simulink model "ex11"  (Simulink 6.3)
settings: Solver=VariableStepDiscrete  StartTime=0.0  StopTime=10.0  RelTol=1e-3
values from neighbouring files (symbols this model uses):
  BitRate = 100000    [ex11sim.m]
  Lc = 7    [ex11sim.m]
libraries: commcnvcod2 x3, commdigbbndpm2 x2, commsink2 x2, commchan3 x1, commrandsrc2 x1, simulink x1
settings Model: LastModifiedBy=lxy  StrictBusMsg=None
settings OptimizationCC: InlineInvariantSignals=on

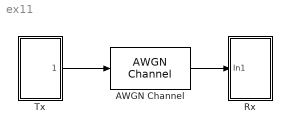
== system ex11 ==
  AWGN Channel : commchan3/AWGN Channel  seed=67  noiseMode="Signal to noise ratio  (Eb/No)"  EbNodB=SNR  EsNodB=10  SNRdB=10  bitsPerSym=1  Ps=1  Tsym=1/BitRate  variance=1
  Rx : Subsystem
  Tx : Subsystem
  wires:
  Tx/1(Signal) -> AWGN Channel/1
  AWGN Channel/1 -> Rx/1(In1)

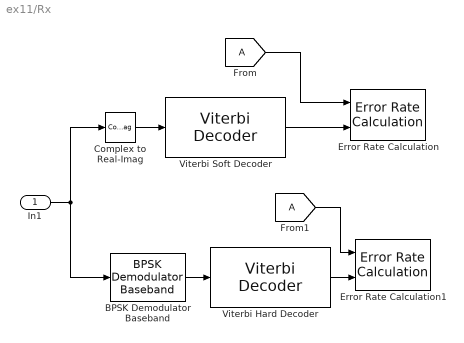
== system ex11/Rx ==
  In1 : Inport
  BPSK Demodulator Baseband : commdigbbndpm2/BPSK Demodulator Baseband  Ph=0  numSamp=1
  Complex to Real-Imag : ComplexToRealImag  Output=Real
  Error Rate Calculation : commsink2/Error Rate Calculation  N=0  st_delay=6*Lc  cp_mode=Entire frame  subframe=[]  PMode=Workspace  WsName=BER2  RsMode2=off  stop=off  numErr=100  maxBits=1e6
  Error Rate Calculation1 : commsink2/Error Rate Calculation  N=0  st_delay=6*Lc  cp_mode=Entire frame  subframe=[]  PMode=Workspace  WsName=BER1  RsMode2=off  stop=off  numErr=100  maxBits=1e6
  Viterbi Hard Decoder : commcnvcod2/Viterbi Decoder  trellis=poly2trellis(Lc, [171 133])  dectype=Hard Decision  nsdecb=4  tbdepth=6*Lc  opmode=Continuous  reset=off  outDataType=double
  Viterbi Soft Decoder : commcnvcod2/Viterbi Decoder  trellis=poly2trellis(Lc, [171 133])  dectype=Unquantized  nsdecb=4  tbdepth=6*Lc  opmode=Continuous  reset=off  outDataType=double
  wires:
  In1/1 -> Complex to Real-Imag/1, BPSK Demodulator Baseband/1
  BPSK Demodulator Baseband/1 -> Viterbi Hard Decoder/1
  Complex to Real-Imag/1 -> Viterbi Soft Decoder/1
  Viterbi Soft Decoder/1 -> Error Rate Calculation/2
  [A] -> Error Rate Calculation/1
  [A] -> Error Rate Calculation1/1
  Viterbi Hard Decoder/1 -> Error Rate Calculation1/2

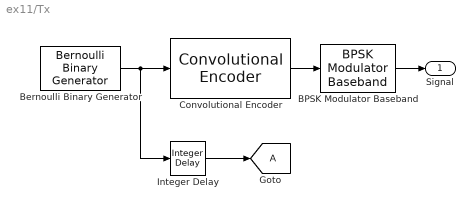
== system ex11/Tx ==
  BPSK Modulator Baseband : commdigbbndpm2/BPSK Modulator Baseband  Ph=0  numSamp=1
  Bernoulli Binary Generator : commrandsrc2/Bernoulli Binary Generator  P=0.5  seed=61  Ts=1/BitRate  frameBased=on  sampPerFrame=BitRate  orient=off  outDataType=double
  Convolutional Encoder : commcnvcod2/Convolutional Encoder  trellis=poly2trellis(Lc, [171 133])  reset=None
  Integer Delay : simulink/Discrete/Integer Delay  vinit=0.0  samptime=-1  NumDelays=6*Lc
  Signal : Outport
  tag scope: A=global
  wires:
  Bernoulli Binary Generator/1 -> Convolutional Encoder/1, Integer Delay/1
  Convolutional Encoder/1 -> BPSK Modulator Baseband/1
  BPSK Modulator Baseband/1 -> Signal/1
  Integer Delay/1 -> [A]
